simulink model "asbQuadcopter"  (R2018b)
settings: Solver=ode3  StartTime=0  StopTime=TFinal  FixedStep=Ts  RelTol=1e-3  EnableMultiTasking=on
undefined symbols (not defined in the file or in its folder): Command, ft, init, m, s, takeOffDuration, Ts, Vehicle
libraries: simulink x16, aerolibconvert2 x4, aerolibanimutils x2, SignalEditorBlockLib x2, environmentLibrary x2, sensorsLibrary x2, aerolibfltsims x2, aerolibutil x2, vrlib x1
settings Model: Creator=The MathWorks, Inc.  LastModifiedBy=The MathWorks, Inc.
settings DataIOCC: LimitDataPoints=on  SaveFormat=Array  SaveOutput=off  SignalLogging=off  DSMLogging=off  SaveTime=off
settings OptimizationCC: BlockReduction=off  BufferReuse=off  LifeSpan=inf
settings DebuggingCC: AlgebraicLoopMsg=none  ParameterPrecisionLossMsg=none  UnconnectedInputMsg=none  UnconnectedOutputMsg=none  UnconnectedLineMsg=none  AllowSymbolicDim=off  LibraryContextMissingDiagnostic=none  SFUnexpectedBacktrackingDiag=warning  SFNoUnconditionalDefaultTransitionDiag=warning  SFExecutionAtInitializationDiag=none
settings HardwareCC: ProdBitPerPointer=32  ProdBitPerSizeT=32  ProdBitPerPtrDiffT=32  ProdLargestAtomicFloat=None  ProdIntDivRoundTo=Undefined  ProdEndianess=Unspecified  ProdWordSize=32  ProdHWDeviceType=32-bit Generic
settings ModelReferenceCC: PropagateSignalLabelsOutOfModel=off
settings SFSimCC: SimUseLocalCustomCode=off
settings RTWCC: RTWUseLocalCustomCode=off
settings CodeAppCC: StateflowObjectComments=on
settings GRTTargetCC: TargetLangStandard=C89/C90 (ANSI)  GeneratePreprocessorConditionals=Disable all
settings ConfigComp: CovMetricSettings=dw  CovHtmlReporting=on  CovSaveCumulativeToWorkspaceVar=on  CovSaveSingleToWorkspaceVar=on  CovExternalEMLEnable=off  CovSFcnEnable=off

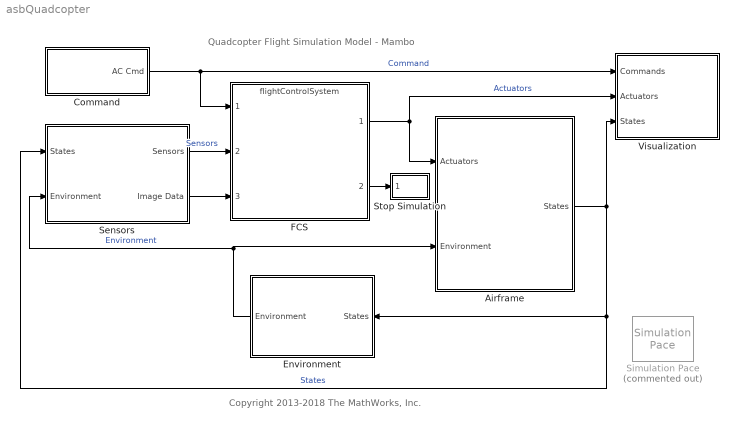
== system asbQuadcopter ==
  note: Quadcopter Flight Simulation Model - Mambo
  note: Copyright 2013-2018 The MathWorks, Inc.
  Airframe : Subsystem  Variant=on
  Command : Subsystem  Variant=on
  Environment : Subsystem  Variant=on
  FCS : ModelReference  ModelNameDialog=flightControlSystem.slx  SimulationMode=Normal  ModelReferenceVersion=1.137
  Sensors : Subsystem  Variant=on
  Simulation Pace : aerolibanimutils/Simulation Pace  Commented=on  SimulationPace=1  SleepMode=MATLAB Thread  OutputPaceError=off  SampleTime=Ts
      settings: AttributesFormatString=%<SimulationPace> sec/sec
  Stop Simulation : Subsystem
  Visualization : Subsystem
  wires:
  Command/1(AC Cmd) -> Visualization/1(Commands), FCS/1  "Command"
  Sensors/1(Sensors) -> FCS/2  "Sensors"
  FCS/1 -> Visualization/2(Actuators), Airframe/1(Actuators)  "Actuators"
  Environment/1(Environment) -> Airframe/2(Environment), Sensors/2(Environment)  "Environment"
  Airframe/1(States) -> Visualization/3(States), Environment/1(States), Sensors/1(States)  "States"
  FCS/2 -> Stop Simulation/1(Flags)
  Sensors/2(Image Data) -> FCS/3

== system asbQuadcopter/Airframe ==
  note: VSS_VEHICLE = 0 will select linear airframe
      | VSS_VEHICLE = 1 will select nonlnear airframe
  Actuators : Inport
  Environment : Inport  Port=2  OutDataTypeStr=Bus: EnvironmentBus
  Linear Airframe : ModelReference  ModelNameDialog=linearAirframe.slx  SimulationMode=Normal  VariantControl=VSS_VEHICLE_LINEAR  ModelReferenceVersion=1.39
  Nonlinear Airframe : ModelReference  ModelNameDialog=nonlinearAirframe.slx  SimulationMode=Normal  VariantControl=VSS_VEHICLE_NONLINEAR  ModelReferenceVersion=1.149
  States : Outport  OutDataTypeStr=Bus: StatesBus

== system asbQuadcopter/Command ==
  note: VSS_COMMAND = 0 will select Signal Editor
      | VSS_COMMAND = 1 will select Joystick + Signal Editor
      | VSS_COMMAND = 2 will select pre-saved data from .mat file
      | VSS_COMMAND = 3 will select pre-saved data from a spreadsheet
  Data : Subsystem  VariantControl=VSS_COMMAND_PRESAVED
  Joystick : Subsystem  VariantControl=VSS_COMMAND_JOYSTICK
  Signal Editor : Subsystem  VariantControl=VSS_COMMAND_SIGEDIT
  Spreadsheet Data : Subsystem  VariantControl=VSS_COMMAND_SPREADSHEET
  AC Cmd : Outport  OutDataTypeStr=Bus: CommandBus

== system asbQuadcopter/Environment ==
  note: VSS_ENVIRONMENT = 0 will select constant environment variables
      | VSS_ENVIRONMENT = 1 will select environment variables depending on position
  States : Inport  OutDataTypeStr=Bus: StatesBus
  Environment (Constant) : environmentLibrary/Environment (Constant)  SystemSampleTime=-1  VariantControl=VSS_ENVIRONMENT_CST
      settings: SourceProductName=Aerospace Blockset  SourceProductBaseCode=AE
  Environment (Variable) : environmentLibrary/Environment (Variable)  SystemSampleTime=-1  VariantControl=VSS_ENVIRONMENT_VARIABLE
      settings: SourceProductName=Aerospace Blockset  SourceProductBaseCode=AE
  Environment : Outport  OutDataTypeStr=Bus: EnvironmentBus

== system asbQuadcopter/Sensors ==
  note: VSS_SENSORS = 0 will select feedthrough sensors
      | VSS_SENSORS = 1 will select dynamics sensors with noise
  States : Inport
  Environment : Inport  Port=2
  Sensors (Dynamics) : sensorsLibrary/Sensors (Dynamics)  SystemSampleTime=-1  VariantControl=VSS_SENSORS_DYNAMICS
      settings: SourceProductName=Aerospace Blockset  SourceProductBaseCode=AE
  Sensors (Feedthrough) : sensorsLibrary/Sensors (Feedthrough)  SystemSampleTime=-1  VariantControl=VSS_SENSORS_FEEDTHROUGH
      settings: SourceProductName=Aerospace Blockset  SourceProductBaseCode=AE
  Sensors : Outport
  Image Data : Outport  Port=2

== system asbQuadcopter/Stop Simulation ==
  Flags : Inport  OutDataTypeStr=uint8
  Compare To Zero : simulink/Logic and Bit Operations/Compare To Zero  relop=>  OutDataTypeStr=boolean
  Flag has been triggered : Assertion
  Logical Operator : Logic  Operator=NOT  AllPortsSameDT=off  OutDataTypeStr=boolean
  wires:
  Flags/1 -> Compare To Zero/1
  Logical Operator/1 -> Flag has been triggered/1
  Compare To Zero/1 -> Logical Operator/1

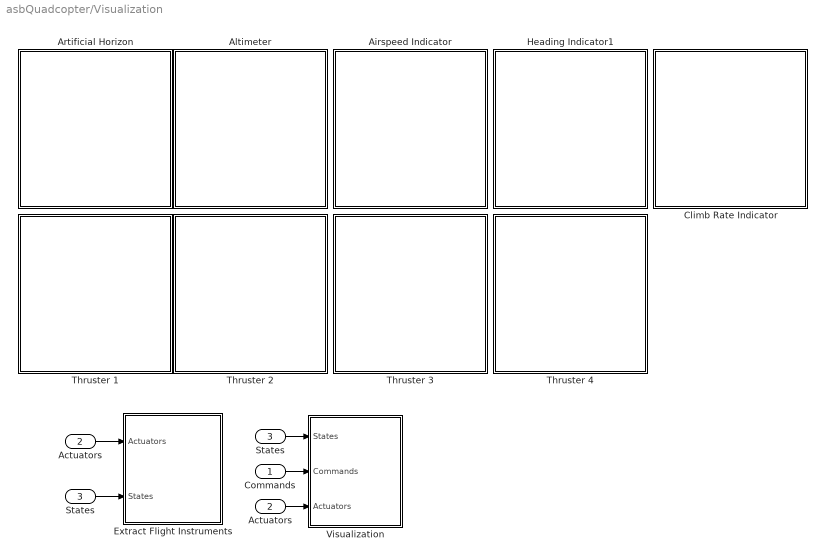
== system asbQuadcopter/Visualization ==
  Commands : Inport
  Actuators : Inport  Port=2
  States : Inport  Port=3
  "Actuators " : InportShadow  Port=2
  Airspeed Indicator : Subsystem  DialogController=aeroblksHMICreateDDGDialog  IsWebBlock=on  mask(MWDashboardBlock){webBlockId=18ef8fab-31e9-4f7d-84d7-de450e3677f8, webBlockType=airspeedindicator, ShowLibInBrowser=on, ShowInitialText=on, HMISrcModelName=asbQuadcopter}
      mask prompts: webBlockId "WebBlock Id"; webBlockType "WebBlock Type"; HMISrcModelName "Source Model"
      mask help: aeroblksHMI:aeroblkhmi:AirspeedIndicatorDialogDesc
      mask Help: eval('asbhmihelp(''airspeedindicator'')');
      mask Display:
      | if strcmp(get_param(bdroot(gcb),'BlockDiagramType'), 'library')
      |  image([(matlabroot) '/toolbox/aeroblks/aeroblks/hmi/icons/AirspeedIndicatorIcon.svg'])
      | end
  Altimeter : Subsystem  DialogController=aeroblksHMICreateDDGDialog  IsWebBlock=on  mask(MWDashboardBlock){webBlockId=100f33d8-dd26-4cf5-9a56-796be033f673, webBlockType=altimeter, ShowLibInBrowser=on, ShowInitialText=on, HMISrcModelName=asbQuadcopter}
      mask prompts: webBlockId "WebBlock Id"; webBlockType "WebBlock Type"; HMISrcModelName "Source Model"
      mask help: aeroblksHMI:aeroblkhmi:AltimeterDialogDesc
      mask Help: eval('asbhmihelp(''altimeter'')');
      mask Display:
      | if strcmp(get_param(bdroot(gcb),'BlockDiagramType'), 'library')
      |  image([(matlabroot) '/toolbox/aeroblks/aeroblks/hmi/icons/AltimeterIcon.svg'])
      | end
  Artificial Horizon : Subsystem  DialogController=aeroblksHMICreateDDGDialog  IsWebBlock=on  mask(MWDashboardBlock){webBlockId=2f185b59-f257-45c3-93d6-8e4e2ebb9412, webBlockType=artificialhorizon, ShowLibInBrowser=on, ShowInitialText=on, HMISrcModelName=asbQuadcopter}
      mask prompts: webBlockId "WebBlock Id"; webBlockType "WebBlock Type"; HMISrcModelName "Source Model"
      mask help: aeroblksHMI:aeroblkhmi:ArtificialHorizonDialogDesc
      mask Help: eval('asbhmihelp(''artificialhorizon'')');
      mask Display:
      | if strcmp(get_param(bdroot(gcb),'BlockDiagramType'), 'library')
      |  image([(matlabroot) '/toolbox/aeroblks/aeroblks/hmi/icons/ArtificialHorizonIcon.svg'])
      | end
  Climb Rate Indicator : Subsystem  DialogController=aeroblksHMICreateDDGDialog  IsWebBlock=on  mask(MWDashboardBlock){webBlockId=01b27fea-40d1-4afa-95b8-217bdf758396, webBlockType=climbindicator, ShowLibInBrowser=on, ShowInitialText=on, HMISrcModelName=asbQuadcopter}
      mask prompts: webBlockId "WebBlock Id"; webBlockType "WebBlock Type"; HMISrcModelName "Source Model"
      mask Help: eval('asbhmihelp(''climbindicator'')');
      mask Display:
      | if strcmp(get_param(bdroot(gcb),'BlockDiagramType'), 'library')
      |  image([(matlabroot) '/toolbox/aeroblks/aeroblks/hmi/icons/ClimbIndicatorIcon.svg'])
      | end
  Extract Flight Instruments : Subsystem
  Heading Indicator1 : Subsystem  DialogController=aeroblksHMICreateDDGDialog  IsWebBlock=on  mask(MWDashboardBlock){webBlockId=349a9895-ae71-4c34-aaf3-8a4b044263fc, webBlockType=headingindicator, ShowLibInBrowser=on, ShowInitialText=on, HMISrcModelName=asbQuadcopter}
      mask prompts: webBlockId "WebBlock Id"; webBlockType "WebBlock Type"; HMISrcModelName "Source Model"
      mask help: aeroblksHMI:aeroblkhmi:HeadingIndicatorDialogDesc
      mask Help: eval('asbhmihelp(''headingindicator'')');
      mask Display:
      | if strcmp(get_param(bdroot(gcb),'BlockDiagramType'), 'library')
      |  image([(matlabroot) '/toolbox/aeroblks/aeroblks/hmi/icons/HeadingIndicatorIcon.svg'])
      | end
  "States " : InportShadow  Port=3
  Thruster 1 : Subsystem  DialogController=aeroblksHMICreateDDGDialog  IsWebBlock=on  mask(MWDashboardBlock){webBlockId=cb5b89b4-9a60-4ffc-8d4b-680aac62b0ad, webBlockType=rpmindicator, ShowLibInBrowser=on, ShowInitialText=on, HMISrcModelName=asbQuadcopter}
      mask prompts: webBlockId "WebBlock Id"; webBlockType "WebBlock Type"; HMISrcModelName "Source Model"
      mask help: aeroblksHMI:aeroblkhmi:RPMIndicatorDialogDesc
      mask Help: eval('asbhmihelp(''rpmindicator'')')
      mask Display:
      | if strcmp(get_param(bdroot(gcb),'BlockDiagramType'), 'library')
      |  image([(matlabroot) '/toolbox/aeroblks/aeroblks/hmi/icons/RPMIndicatorIcon.svg'])
      | end
  Thruster 2 : Subsystem  DialogController=aeroblksHMICreateDDGDialog  IsWebBlock=on  mask(MWDashboardBlock){webBlockId=f0cf643f-3686-4bab-9794-ec5ca9f0526b, webBlockType=rpmindicator, ShowLibInBrowser=on, ShowInitialText=on, HMISrcModelName=asbQuadcopter}
      mask prompts: webBlockId "WebBlock Id"; webBlockType "WebBlock Type"; HMISrcModelName "Source Model"
      mask help: aeroblksHMI:aeroblkhmi:RPMIndicatorDialogDesc
      mask Help: eval('asbhmihelp(''rpmindicator'')')
      mask Display:
      | if strcmp(get_param(bdroot(gcb),'BlockDiagramType'), 'library')
      |  image([(matlabroot) '/toolbox/aeroblks/aeroblks/hmi/icons/RPMIndicatorIcon.svg'])
      | end
  Thruster 3 : Subsystem  DialogController=aeroblksHMICreateDDGDialog  IsWebBlock=on  mask(MWDashboardBlock){webBlockId=fde82f48-64f7-4e22-ac0c-568ccc998d28, webBlockType=rpmindicator, ShowLibInBrowser=on, ShowInitialText=on, HMISrcModelName=asbQuadcopter}
      mask prompts: webBlockId "WebBlock Id"; webBlockType "WebBlock Type"; HMISrcModelName "Source Model"
      mask help: aeroblksHMI:aeroblkhmi:RPMIndicatorDialogDesc
      mask Help: eval('asbhmihelp(''rpmindicator'')')
      mask Display:
      | if strcmp(get_param(bdroot(gcb),'BlockDiagramType'), 'library')
      |  image([(matlabroot) '/toolbox/aeroblks/aeroblks/hmi/icons/RPMIndicatorIcon.svg'])
      | end
  Thruster 4 : Subsystem  DialogController=aeroblksHMICreateDDGDialog  IsWebBlock=on  mask(MWDashboardBlock){webBlockId=9efa2ed4-730f-4ead-a19e-56fcb1fb4e55, webBlockType=rpmindicator, ShowLibInBrowser=on, ShowInitialText=on, HMISrcModelName=asbQuadcopter}
      mask prompts: webBlockId "WebBlock Id"; webBlockType "WebBlock Type"; HMISrcModelName "Source Model"
      mask help: aeroblksHMI:aeroblkhmi:RPMIndicatorDialogDesc
      mask Help: eval('asbhmihelp(''rpmindicator'')')
      mask Display:
      | if strcmp(get_param(bdroot(gcb),'BlockDiagramType'), 'library')
      |  image([(matlabroot) '/toolbox/aeroblks/aeroblks/hmi/icons/RPMIndicatorIcon.svg'])
      | end
  Visualization : Subsystem  Variant=on
  wires:
  Actuators/1 -> Extract Flight Instruments/1(Actuators)
  States/1 -> Extract Flight Instruments/2(States)
  Commands/1 -> Visualization/2(Commands)
  "Actuators "/1 -> Visualization/3(Actuators)
  "States "/1 -> Visualization/1(States)

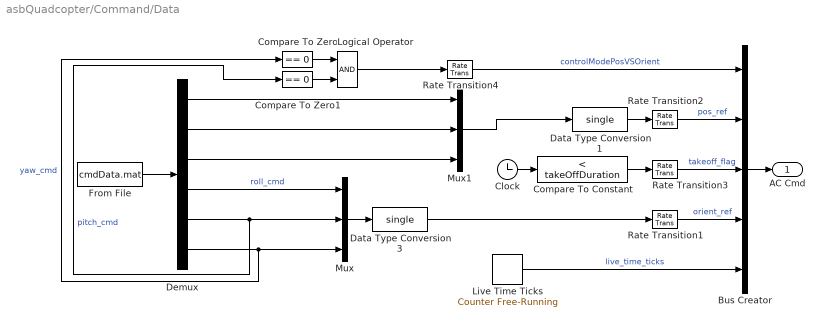
== system asbQuadcopter/Command/Data ==
  Bus Creator : BusCreator  Inputs=5  OutDataTypeStr=Bus: CommandBus  NonVirtualBus=on
  Clock : Clock
  Compare To Constant : simulink/Logic and Bit Operations/Compare To Constant  relop=<  const=takeOffDuration  OutDataTypeStr=boolean
  Compare To Zero : simulink/Logic and Bit Operations/Compare To Zero  relop===  OutDataTypeStr=boolean
  Compare To Zero1 : simulink/Logic and Bit Operations/Compare To Zero  relop===  OutDataTypeStr=boolean
  Data Type Conversion1 : DataTypeConversion  OutDataTypeStr=single
  Data Type Conversion3 : DataTypeConversion  OutDataTypeStr=single
  Demux : Demux  Outputs=6
  From File : FromFile  FileName=cmdData.mat  SampleTime=Ts
  Live Time Ticks : simulink/Sources/Counter Free-Running  NumBits=32  tsamp=Ts
  Logical Operator : Logic  IconShape=distinctive  AllPortsSameDT=off  OutDataTypeStr=boolean
  Mux : Mux  Inputs=3
  Mux1 : Mux  Inputs=3
  Rate Transition{1..4} (4 alike) : RateTransition  OutPortSampleTime=Ts
  AC Cmd : Outport  OutDataTypeStr=Bus: CommandBus
  wires:
  Demux/4 -> Mux/1  "roll_cmd"
  Demux/5 -> Mux/2, Compare To Zero1/1  "pitch_cmd"
  Demux/6 -> Compare To Zero/1, Mux/3  "yaw_cmd"
  From File/1 -> Demux/1
  Logical Operator/1 -> Rate Transition4/1
  Rate Transition1/1 -> Bus Creator/4  "orient_ref"
  Rate Transition2/1 -> Bus Creator/2  "pos_ref"
  Demux/3 -> Mux1/3
  Mux/1 -> Data Type Conversion3/1
  Data Type Conversion1/1 -> Rate Transition2/1
  Demux/1 -> Mux1/1
  Compare To Zero1/1 -> Logical Operator/2
  Compare To Zero/1 -> Logical Operator/1
  Mux1/1 -> Data Type Conversion1/1
  Clock/1 -> Compare To Constant/1
  Rate Transition4/1 -> Bus Creator/1  "controlModePosVSOrient"
  Data Type Conversion3/1 -> Rate Transition1/1
  Demux/2 -> Mux1/2
  Compare To Constant/1 -> Rate Transition3/1
  Rate Transition3/1 -> Bus Creator/3  "takeoff_flag"
  Live Time Ticks/1 -> Bus Creator/5  "live_time_ticks"
  Bus Creator/1 -> AC Cmd/1

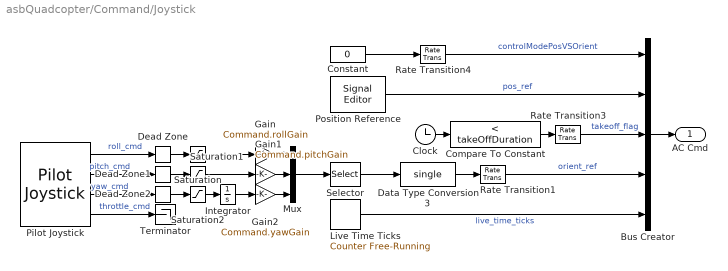
== system asbQuadcopter/Command/Joystick ==
  Bus Creator : BusCreator  Inputs=5  OutDataTypeStr=Bus: CommandBus  NonVirtualBus=on
  Clock : Clock
  Compare To Constant : simulink/Logic and Bit Operations/Compare To Constant  relop=<  const=takeOffDuration  OutDataTypeStr=boolean
  Constant : Constant  Value=0  OutDataTypeStr=boolean
  Data Type Conversion3 : DataTypeConversion  OutDataTypeStr=single
  Dead Zone : DeadZone  LowerValue=Command.rollDeadZoneStart  UpperValue=Command.rollDeadZoneEnd  SaturateOnIntegerOverflow=on
  Dead Zone1 : DeadZone  LowerValue=Command.pitchDeadZoneStart  UpperValue=Command.pitchDeadZoneEnd  SaturateOnIntegerOverflow=on
  Dead Zone2 : DeadZone  LowerValue=Command.yawDeadZoneStart  UpperValue=Command.yawDeadZoneEnd  SaturateOnIntegerOverflow=on
  Gain : Gain  Gain=Command.rollGain
  Gain1 : Gain  Gain=Command.pitchGain
  Gain2 : Gain  Gain=Command.yawGain
  Integrator : Integrator
  Live Time Ticks : simulink/Sources/Counter Free-Running  NumBits=32  tsamp=Ts
  Mux : Mux  Inputs=3
  Pilot Joystick : aerolibanimutils/Pilot Joystick  JoystickID=Joystick1  OutputConfiguration=FourAxis  SampleTime=Ts
  Position Reference : SignalEditorBlockLib/Signal Editor  FileName=positionRef.mat  ActiveScenario=Group1  ActiveSignal=XYZ  IsBus=off  OutputBusObjectStr=Bus: BusObject  SampleTime=Ts  Interpolate=off  ZeroCross=off  OutputAfterFinalValue=Setting to zero  Unit=inherit
  Rate Transition1 : RateTransition  OutPortSampleTime=Ts
  Rate Transition3 : RateTransition  OutPortSampleTime=Ts
  Rate Transition4 : RateTransition  OutPortSampleTime=Ts
  Saturation : Saturate  UpperLimit=Command.rollSatUpper  LowerLimit=Command.rollSatLower
  Saturation1 : Saturate  UpperLimit=Command.pitchSatUpper  LowerLimit=Command.pitchSatLower
  Saturation2 : Saturate  UpperLimit=Command.yawSatUpper  LowerLimit=Command.yawSatLower
  Selector : Selector  InputPortWidth=3  IndexOptions=Index vector (dialog)  Indices=[3 2 1]  OutputSizes=1
  Terminator : Terminator
  AC Cmd : Outport  OutDataTypeStr=Bus: CommandBus
  wires:
  Pilot Joystick/4 -> Terminator/1  "throttle_cmd"
  Pilot Joystick/1 -> Dead Zone/1  "roll_cmd"
  Bus Creator/1 -> AC Cmd/1
  Constant/1 -> Rate Transition4/1
  Rate Transition1/1 -> Bus Creator/4  "orient_ref"
  Position Reference/1 -> Bus Creator/2  "pos_ref"
  Mux/1 -> Selector/1
  Compare To Constant/1 -> Rate Transition3/1
  Clock/1 -> Compare To Constant/1
  Rate Transition4/1 -> Bus Creator/1  "controlModePosVSOrient"
  Data Type Conversion3/1 -> Rate Transition1/1
  Pilot Joystick/2 -> Dead Zone1/1  "pitch_cmd"
  Rate Transition3/1 -> Bus Creator/3  "takeoff_flag"
  Live Time Ticks/1 -> Bus Creator/5  "live_time_ticks"
  Selector/1 -> Data Type Conversion3/1
  Dead Zone/1 -> Saturation/1
  Saturation/1 -> Gain/1
  Gain/1 -> Mux/1
  Dead Zone1/1 -> Saturation1/1
  Saturation1/1 -> Gain1/1
  Gain1/1 -> Mux/2
  Dead Zone2/1 -> Saturation2/1
  Saturation2/1 -> Integrator/1
  Gain2/1 -> Mux/3
  Pilot Joystick/3 -> Dead Zone2/1  "yaw_cmd"
  Integrator/1 -> Gain2/1

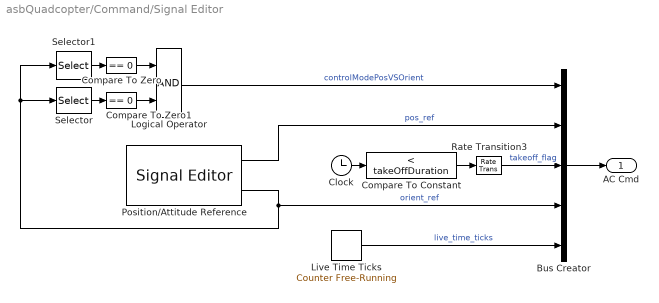
== system asbQuadcopter/Command/Signal Editor ==
  Bus Creator : BusCreator  Inputs=5  OutDataTypeStr=Bus: CommandBus  NonVirtualBus=on
  Clock : Clock
  Compare To Constant : simulink/Logic and Bit Operations/Compare To Constant  relop=<  const=takeOffDuration  OutDataTypeStr=boolean
  Compare To Zero : simulink/Logic and Bit Operations/Compare To Zero  relop===  OutDataTypeStr=boolean
  Compare To Zero1 : simulink/Logic and Bit Operations/Compare To Zero  relop===  OutDataTypeStr=boolean
  Live Time Ticks : simulink/Sources/Counter Free-Running  NumBits=32  tsamp=Ts
  Logical Operator : Logic  AllPortsSameDT=off  OutDataTypeStr=boolean
  Position/Attitude Reference : SignalEditorBlockLib/Signal Editor  FileName=positionAttitudeRef.mat  ActiveScenario=Hover  ActiveSignal=XYZ  IsBus=off  OutputBusObjectStr=Bus: BusObject  SampleTime=Ts  Interpolate=off  ZeroCross=off  OutputAfterFinalValue=Holding final value  Unit=inherit
  Rate Transition3 : RateTransition  OutPortSampleTime=Ts
  Selector : Selector  InputPortWidth=3  IndexOptions=Index vector (dialog)  Indices=2  OutputSizes=1
  Selector1 : Selector  InputPortWidth=3  IndexOptions=Index vector (dialog)  Indices=3  OutputSizes=1
  AC Cmd : Outport  OutDataTypeStr=Bus: CommandBus
  wires:
  Bus Creator/1 -> AC Cmd/1
  Position/Attitude Reference/2 -> Bus Creator/4, Selector1/1, Selector/1  "orient_ref"
  Compare To Zero/1 -> Logical Operator/1
  Compare To Zero1/1 -> Logical Operator/2
  Logical Operator/1 -> Bus Creator/1  "controlModePosVSOrient"
  Position/Attitude Reference/1 -> Bus Creator/2  "pos_ref"
  Clock/1 -> Compare To Constant/1
  Compare To Constant/1 -> Rate Transition3/1
  Rate Transition3/1 -> Bus Creator/3  "takeoff_flag"
  Live Time Ticks/1 -> Bus Creator/5  "live_time_ticks"
  Selector/1 -> Compare To Zero1/1
  Selector1/1 -> Compare To Zero/1

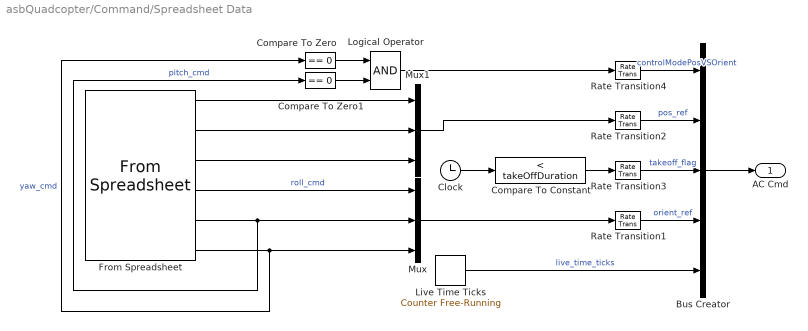
== system asbQuadcopter/Command/Spreadsheet Data ==
  Bus Creator : BusCreator  Inputs=5  OutDataTypeStr=Bus: CommandBus  NonVirtualBus=on
  Clock : Clock
  Compare To Constant : simulink/Logic and Bit Operations/Compare To Constant  relop=<  const=takeOffDuration  OutDataTypeStr=boolean
  Compare To Zero : simulink/Logic and Bit Operations/Compare To Zero  relop===  OutDataTypeStr=boolean
  Compare To Zero1 : simulink/Logic and Bit Operations/Compare To Zero  relop===  OutDataTypeStr=boolean
  From Spreadsheet : FromSpreadsheet  FileName=cmdData.xlsx  SheetName=data  OutDataTypeStr=single  SampleTime=Ts
  Live Time Ticks : simulink/Sources/Counter Free-Running  NumBits=32  tsamp=Ts
  Logical Operator : Logic  IconShape=distinctive  AllPortsSameDT=off  OutDataTypeStr=boolean
  Mux : Mux  Inputs=3
  Mux1 : Mux  Inputs=3
  Rate Transition{1..4} (4 alike) : RateTransition  OutPortSampleTime=Ts
  AC Cmd : Outport  OutDataTypeStr=Bus: CommandBus
  wires:
  Bus Creator/1 -> AC Cmd/1
  From Spreadsheet/4 -> Mux/1  "roll_cmd"
  From Spreadsheet/6 -> Mux/3, Compare To Zero/1  "yaw_cmd"
  Logical Operator/1 -> Rate Transition4/1
  Rate Transition1/1 -> Bus Creator/4  "orient_ref"
  Rate Transition2/1 -> Bus Creator/2  "pos_ref"
  From Spreadsheet/3 -> Mux1/3
  Mux1/1 -> Rate Transition2/1
  From Spreadsheet/1 -> Mux1/1
  Compare To Zero1/1 -> Logical Operator/2
  Compare To Zero/1 -> Logical Operator/1
  Compare To Constant/1 -> Rate Transition3/1
  Clock/1 -> Compare To Constant/1
  Rate Transition4/1 -> Bus Creator/1  "controlModePosVSOrient"
  Mux/1 -> Rate Transition1/1
  From Spreadsheet/5 -> Mux/2, Compare To Zero1/1  "pitch_cmd"
  From Spreadsheet/2 -> Mux1/2
  Rate Transition3/1 -> Bus Creator/3  "takeoff_flag"
  Live Time Ticks/1 -> Bus Creator/5  "live_time_ticks"

== system asbQuadcopter/Visualization/Airspeed Indicator ==

== system asbQuadcopter/Visualization/Altimeter ==

== system asbQuadcopter/Visualization/Artificial Horizon ==

== system asbQuadcopter/Visualization/Climb Rate Indicator ==

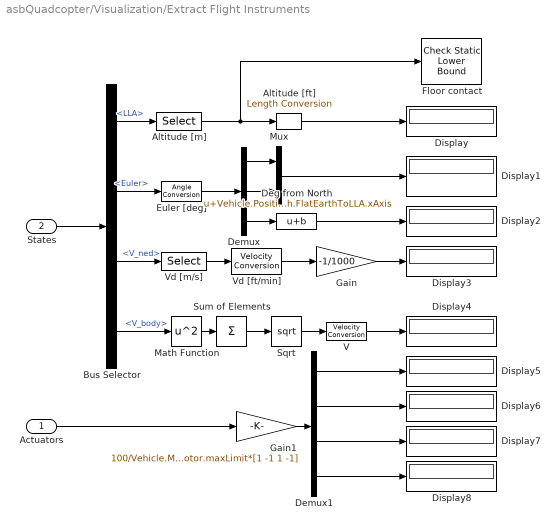
== system asbQuadcopter/Visualization/Extract Flight Instruments ==
  Actuators : Inport
  States : Inport  Port=2
  Altitude [ft] : aerolibconvert2/Length Conversion  IU=m  OU=ft
  Altitude [m] : Selector  InputPortWidth=3  IndexOptions=Index vector (dialog)  Indices=[3]  OutputSizes=1
  Bus Selector : BusSelector  OutputSignals=LLA,Euler,V_ned,V_body
  Deg from North : Bias  Bias=Vehicle.PositionOnEarth.FlatEarthToLLA.xAxis
  Demux : Demux  Outputs=3
  Demux1 : Demux
  Display{,1..8} (9 alike) : Display
  Euler [deg] : aerolibconvert2/Angle Conversion  IU=rad  OU=deg
  Floor contact : simulink/Model Verification/Check Static  Lower Bound  Description=init.posLLA(3) <= u  min=init.posLLA(3)  min_included=on  enabled=on  stopWhenAssertionFail=on  export=off  icon=graphic
      settings: SourceProductName=Simulink
  Gain : Gain  Gain=-1/1000
  Gain1 : Gain  Gain=100/Vehicle.Motor.maxLimit*[1 -1 1 -1]
  Math Function : Math  Operator=square  SaturateOnIntegerOverflow=on
  Mux : Mux  Inputs=2
  Sqrt : Sqrt  SaturateOnIntegerOverflow=on
  Sum of Elements : Sum  Inputs=+
  V : aerolibconvert2/Velocity Conversion  IU=m/s  OU=kts
  Vd [ft/min] : aerolibconvert2/Velocity Conversion  IU=m/s  OU=ft/min
  Vd [m/s] : Selector  InputPortWidth=3  IndexOptions=Index vector (dialog)  Indices=[3]  OutputSizes=1
  wires:
  Bus Selector/1 -> Altitude [m]/1  "<LLA>"
  Altitude [m]/1 -> Floor contact/1, Altitude [ft]/1
  States/1 -> Bus Selector/1
  Altitude [ft]/1 -> Display/1
  Bus Selector/2 -> Euler [deg]/1  "<Euler>"
  Euler [deg]/1 -> Demux/1
  Demux/1 -> Mux/1
  Demux/2 -> Mux/2
  Mux/1 -> Display1/1
  Deg from North/1 -> Display2/1
  Bus Selector/3 -> Vd [m/s]/1  "<V_ned>"
  Vd [m/s]/1 -> Vd [ft/min]/1
  Vd [ft/min]/1 -> Gain/1
  Gain/1 -> Display3/1
  Math Function/1 -> Sum of Elements/1
  Sum of Elements/1 -> Sqrt/1
  Bus Selector/4 -> Math Function/1  "<V_body>"
  Sqrt/1 -> V/1
  V/1 -> Display4/1
  Gain1/1 -> Demux1/1
  Demux1/1 -> Display5/1
  Demux1/2 -> Display6/1
  Demux1/3 -> Display7/1
  Demux1/4 -> Display8/1
  Actuators/1 -> Gain1/1
  Demux/3 -> Deg from North/1

== system asbQuadcopter/Visualization/Heading Indicator1 ==

== system asbQuadcopter/Visualization/Thruster 1 ==

== system asbQuadcopter/Visualization/Thruster 2 ==

== system asbQuadcopter/Visualization/Thruster 3 ==

== system asbQuadcopter/Visualization/Thruster 4 ==

== system asbQuadcopter/Visualization/Visualization ==
  note: VSS_VISUALIZATION = 0 will select scopes as means to visualie variables/states
      | VSS_VISUALIZATION = 1 will send select states in a variable to the workspace
      | VSS_VISUALIZATION = 2 will use FlightGear as visualization
      | VSS_VISUALIZATION = 3 will use a Simulink 3D interface
  States : Inport  OutDataTypeStr=Bus: StatesBus
  Commands : Inport  Port=2  OutDataTypeStr=Bus: CommandBus
  Actuators : Inport  Port=3
  FlightGear : Subsystem  VariantControl=VSS_VISUALIZATION_FLIGHTGEAR
      mask init:
      | visualizationFlightGearVars;
  Scopes : Subsystem  VariantControl=VSS_VISUALIZATION_SCOPES
  Simulink 3D : Subsystem  VariantControl=VSS_VISUALIZATION_SL3D
      mask init:
      | visualizationFlightGearVars;
  Workspace : Subsystem  VariantControl=VSS_VISUALIZATION_WORKSPACE

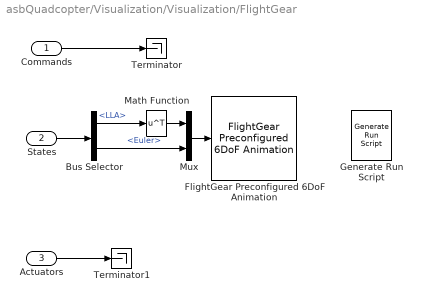
== system asbQuadcopter/Visualization/Visualization/FlightGear ==
  Commands : Inport
  States : Inport  Port=2
  Actuators : Inport  Port=3
  Bus Selector : BusSelector  OutputSignals=LLA,Euler
  FlightGear Preconfigured 6DoF Animation : aerolibfltsims/FlightGear Preconfigured 6DoF Animation  xFlightGearVersion=v2017.3  DestinationIpAddress=127.0.0.1  DestinationPort=Visualization.FlightGear.SixDOF.destinationPort  SampleTime=Ts
      settings: SourceProductName=Aerospace Blockset
  Generate Run Script : aerolibfltsims/Generate Run Script  Architecture=Default  dataFlow=Send  GeometryModelName=Model  AirportId=KSFO  RunwayId=10L  InitialAltitude=Visualization.FlightGear.generateRunScript.initialAltitude  InitialHeading=Visualization.FlightGear.generateRunScript.initialHeading  OffsetDistance=Visualization.FlightGear.generateRunScript.offsetDistance  OffsetAzimuth=Visualization.FlightGear.generateRunScript.offsetAzimuth  InstallScenery=off  DisableShaders=off  OriginAddress=127.0.0.1  DestinationPort=Visualization.FlightGear.generateRunScript.destinationPort  OriginPort=5505  LocalAddress=127.0.0.1  OutputFileName=runfg.bat  FlightGearBaseDirectory=C:\Program Files\FlightGear
  Math Function : Math  Operator=transpose  SaturateOnIntegerOverflow=on
  Mux : Mux  Inputs=2
  Terminator : Terminator
  Terminator1 : Terminator
  wires:
  States/1 -> Bus Selector/1
  Bus Selector/2 -> Mux/2  "<Euler>"
  Mux/1 -> FlightGear Preconfigured 6DoF Animation/1
  Commands/1 -> Terminator/1
  Actuators/1 -> Terminator1/1
  Bus Selector/1 -> Math Function/1  "<LLA>"
  Math Function/1 -> Mux/1

== system asbQuadcopter/Visualization/Visualization/Scopes ==
  Commands : Inport
  States : Inport  Port=2
  Actuators : Inport  Port=3
  Bus Creator : BusCreator  Inputs=2
  Bus Selector : BusSelector  OutputSignals=States.V_body,States.Euler,States.X_ned
  Euler : Scope
  Terminator1 : Terminator
  V_body : Scope
  X_ned : Scope
  wires:
  Commands/1 -> Bus Creator/1  "Commands"
  States/1 -> Bus Creator/2  "States"
  Bus Creator/1 -> Bus Selector/1
  Bus Selector/1 -> V_body/1  "<V_body>"
  Bus Selector/2 -> Euler/1  "<Euler>"
  Bus Selector/3 -> X_ned/1  "<X_ned>"
  Actuators/1 -> Terminator1/1

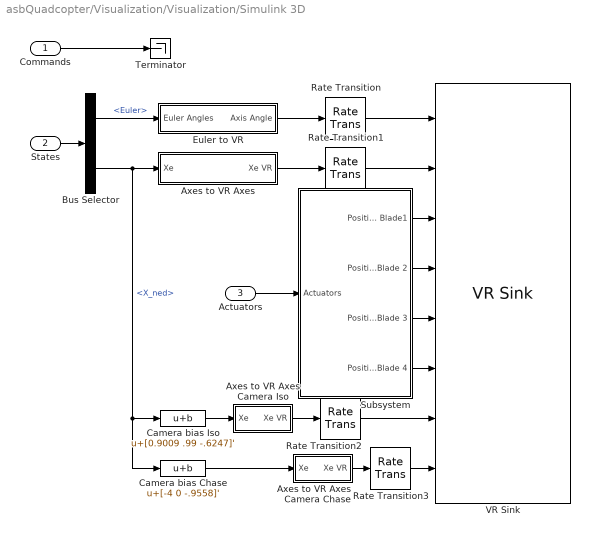
== system asbQuadcopter/Visualization/Visualization/Simulink 3D ==
  Commands : Inport
  States : Inport  Port=2
  Actuators : Inport  Port=3
  Axes to VR Axes : Subsystem
  Axes to VR Axes Camera Chase : Subsystem
  Axes to VR Axes Camera Iso : Subsystem
  Bus Selector : BusSelector  OutputSignals=Euler,X_ned
  Camera bias Chase : Bias  Bias=[-4 0 -.9558]'
  Camera bias Iso : Bias  Bias=[0.9009 .99 -.6247]'
  Euler to VR : Subsystem
  Rate Transition{,1..3} (4 alike) : RateTransition
  Subsystem : Subsystem
  Terminator : Terminator
  VR Sink : vrlib/VR Sink  InstantiateOnLoad=on  SampleTime=12*Ts  ViewEnable=on  RemoteChange=off  RemoteView=off  FieldsWritten=QuadBody.rotation.4.1.1.double#QuadBody.translation.3.1.1.double#Blade1.rotation.4.1.1.double#Blade3.rotation.4.1.1.double#Blade2.rotation.4.1.1.double#Blade4.rotation.4.1.1.double#IsoNoRotation.position.3.1.1.double#OnQuadNoRotation.position.3.1.1.double  WorldFileName=asbQuadcopterWorld.wrl  AutoView=on  VideoDimensions=[]  AllowVariableSize=off  FigureProperties="{'Position', 'Name', 'Viewpoint', 'CameraBound', 'CameraDirection', 'CameraPosition', 'CameraUpVector', 'ZoomFactor', 'Antialiasing', 'Headlight', 'Lighting', 'NavPanel', 'Sound', 'StatusBar', 'Stereo3D', 'Stereo3DCameraOffset', 'Stereo3DHIT', 'ToolBar', 'Textures', 'Transparency', 'Triad', 'Wireframe', 'NavZones', 'NavMode', 'NavSpeed', 'CaptureFileFormat', 'CaptureFileName', 'Record2DCompressMethod', 'Record2DCompressQuality', 'Record2D', 'Record2DFileName', 'Record2DFPS'; [5.0000000000000000e+00   1.0200000000000000e+02   5.7600000000000000e+02   3.5000000000000000e+02], '', 'Isometric', 'on', [0.0000000000000000e+00   0.0000000000000000e+00  -1.0000000000000000e+00], [0.0000000000000000e+00   0.0000000000000000e+00   0.0000000000000000e+00], [0.0000000000000000e+00   1.0000000000000000e+00   0.0000000000000000e+00], [1.0000000000000000e+00], 'on', 'on', 'on', 'halfbar', 'on', 'on', 'off', [1.0000000149011612e-01], [0.0000000000000000e+00], 'on', 'on', 'on', 'none', 'off', 'off', 'fly', 'normal', 'tif', '%f_anim_%n.tif', 'auto', [7.5000000000000000e+01], 'off', '%f_anim_%n.avi', 'auto'}"
      settings: SourceProductBaseCode=VR
  wires:
  Commands/1 -> Terminator/1
  Euler to VR/1(Axis Angle) -> Rate Transition/1
  Axes to VR Axes/1(Xe VR) -> Rate Transition1/1
  Bus Selector/1 -> Euler to VR/1(Euler Angles)  "<Euler>"
  Bus Selector/2 -> Camera bias Chase/1, Camera bias Iso/1, Axes to VR Axes/1(Xe)  "<X_ned>"
  States/1 -> Bus Selector/1
  Actuators/1 -> Subsystem/1(Actuators)
  Axes to VR Axes Camera Iso/1(Xe VR) -> Rate Transition2/1
  Camera bias Iso/1 -> Axes to VR Axes Camera Iso/1(Xe)
  Rate Transition/1 -> VR Sink/1
  Rate Transition1/1 -> VR Sink/2
  Subsystem/1(Position Blade1) -> VR Sink/3
  Subsystem/2(Position Blade 2) -> VR Sink/4
  Subsystem/3(Position Blade 3) -> VR Sink/5
  Subsystem/4(Position Blade 4) -> VR Sink/6
  Rate Transition2/1 -> VR Sink/7
  Axes to VR Axes Camera Chase/1(Xe VR) -> Rate Transition3/1
  Rate Transition3/1 -> VR Sink/8
  Camera bias Chase/1 -> Axes to VR Axes Camera Chase/1(Xe)

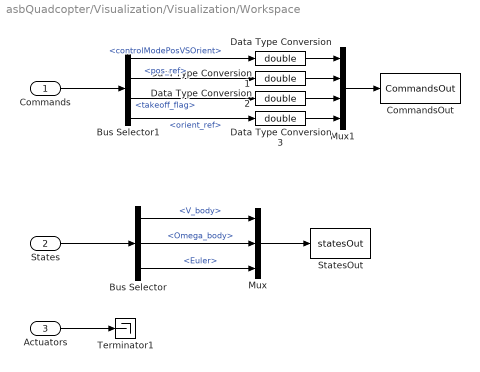
== system asbQuadcopter/Visualization/Visualization/Workspace ==
  Commands : Inport
  States : Inport  Port=2
  Actuators : Inport  Port=3
  Bus Selector : BusSelector  OutputSignals=V_body,Omega_body,Euler
  Bus Selector1 : BusSelector  OutputSignals=controlModePosVSOrient,pos_ref,takeoff_flag,orient_ref
  CommandsOut : ToWorkspace  VariableName=CommandsOut  SaveFormat=Structure With Time  SampleTime=-1
  Data Type Conversion{,1..3} (4 alike) : DataTypeConversion  OutDataTypeStr=double
  Mux : Mux  Inputs=3
  Mux1 : Mux
  StatesOut : ToWorkspace  VariableName=statesOut  SaveFormat=Structure With Time  SampleTime=-1
  Terminator1 : Terminator
  wires:
  States/1 -> Bus Selector/1
  Bus Selector/2 -> Mux/2  "<Omega_body>"
  Bus Selector/3 -> Mux/3  "<Euler>"
  Bus Selector/1 -> Mux/1  "<V_body>"
  Mux/1 -> StatesOut/1
  Commands/1 -> Bus Selector1/1
  Bus Selector1/2 -> Data Type Conversion1/1  "<pos_ref>"
  Bus Selector1/1 -> Data Type Conversion/1  "<controlModePosVSOrient>"
  Mux1/1 -> CommandsOut/1
  Bus Selector1/4 -> Data Type Conversion3/1  "<orient_ref>"
  Bus Selector1/3 -> Data Type Conversion2/1  "<takeoff_flag>"
  Actuators/1 -> Terminator1/1
  Data Type Conversion/1 -> Mux1/1
  Data Type Conversion1/1 -> Mux1/2
  Data Type Conversion2/1 -> Mux1/3
  Data Type Conversion3/1 -> Mux1/4

== system asbQuadcopter/Visualization/Visualization/Simulink 3D/Axes to VR Axes ==
  Xe : Inport
  Demux : Demux  Outputs=3
  Mux : Mux  Inputs=3
  rad-->deg1 : Gain  Gain=-1  SaturateOnIntegerOverflow=on  OutDataTypeStr=Inherit: Same as input  ParamDataTypeStr=Inherit: Same as input
  Xe VR : Outport
  wires:
  Xe/1 -> Demux/1
  Demux/1 -> Mux/1
  Demux/3 -> rad-->deg1/1
  Mux/1 -> Xe VR/1
  rad-->deg1/1 -> Mux/2
  Demux/2 -> Mux/3

== system asbQuadcopter/Visualization/Visualization/Simulink 3D/Axes to VR Axes Camera Chase ==
  Xe : Inport
  Demux : Demux  Outputs=3
  Mux : Mux  Inputs=3
  rad-->deg1 : Gain  Gain=-1  SaturateOnIntegerOverflow=on  OutDataTypeStr=Inherit: Same as input  ParamDataTypeStr=Inherit: Same as input
  Xe VR : Outport
  wires:
  Xe/1 -> Demux/1
  Demux/1 -> Mux/1
  Demux/3 -> rad-->deg1/1
  Mux/1 -> Xe VR/1
  rad-->deg1/1 -> Mux/2
  Demux/2 -> Mux/3

== system asbQuadcopter/Visualization/Visualization/Simulink 3D/Axes to VR Axes Camera Iso ==
  Xe : Inport
  Demux : Demux  Outputs=3
  Mux : Mux  Inputs=3
  rad-->deg1 : Gain  Gain=-1  SaturateOnIntegerOverflow=on  OutDataTypeStr=Inherit: Same as input  ParamDataTypeStr=Inherit: Same as input
  Xe VR : Outport
  wires:
  Demux/2 -> Mux/3
  rad-->deg1/1 -> Mux/2
  Mux/1 -> Xe VR/1
  Demux/3 -> rad-->deg1/1
  Demux/1 -> Mux/1
  Xe/1 -> Demux/1

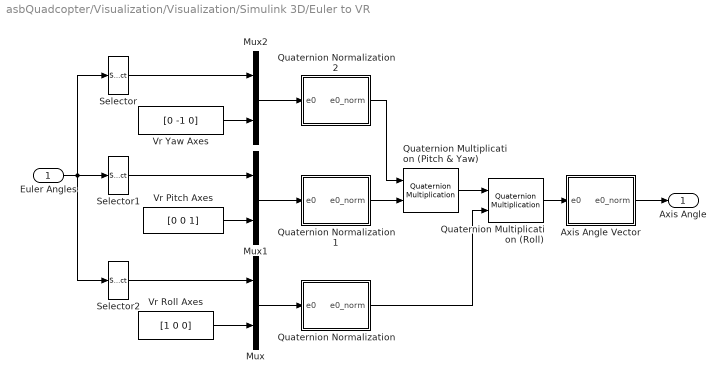
== system asbQuadcopter/Visualization/Visualization/Simulink 3D/Euler to VR ==
  Euler Angles : Inport
  Axis Angle Vector : Subsystem
  Mux : Mux  Inputs=2
  Mux1 : Mux  Inputs=2
  Mux2 : Mux  Inputs=2
  Quaternion Multiplication (Pitch & Yaw) : aerolibutil/Quaternion Multiplication
  Quaternion Multiplication (Roll) : aerolibutil/Quaternion Multiplication
  Quaternion Normalization : Subsystem
  Quaternion Normalization1 : Subsystem
  Quaternion Normalization2 : Subsystem
  Selector : Selector  InputPortWidth=3  IndexOptions=Index vector (dialog)  Indices=[3]  OutputSizes=1
  Selector1 : Selector  InputPortWidth=3  IndexOptions=Index vector (dialog)  Indices=[2]  OutputSizes=1
  Selector2 : Selector  InputPortWidth=3  IndexOptions=Index vector (dialog)  Indices=[1]  OutputSizes=1
  Vr Pitch Axes : Constant  Value=[0 0 1]
  Vr Roll Axes : Constant  Value=[1 0 0]
  Vr Yaw Axes : Constant  Value=[0 -1 0]
  Axis Angle : Outport
  wires:
  Quaternion Multiplication (Roll)/1 -> Axis Angle Vector/1(e0)
  Axis Angle Vector/1(e0_norm) -> Axis Angle/1
  Quaternion Normalization/1(e0_norm) -> Quaternion Multiplication (Roll)/2
  Quaternion Normalization2/1(e0_norm) -> Quaternion Multiplication (Pitch & Yaw)/1
  Quaternion Normalization1/1(e0_norm) -> Quaternion Multiplication (Pitch & Yaw)/2
  Mux2/1 -> Quaternion Normalization2/1(e0)
  Mux1/1 -> Quaternion Normalization1/1(e0)
  Mux/1 -> Quaternion Normalization/1(e0)
  Selector/1 -> Mux2/1
  Vr Yaw Axes/1 -> Mux2/2
  Selector1/1 -> Mux1/1
  Vr Pitch Axes/1 -> Mux1/2
  Selector2/1 -> Mux/1
  Vr Roll Axes/1 -> Mux/2
  Euler Angles/1 -> Selector2/1, Selector1/1, Selector/1
  Quaternion Multiplication (Pitch & Yaw)/1 -> Quaternion Multiplication (Roll)/1

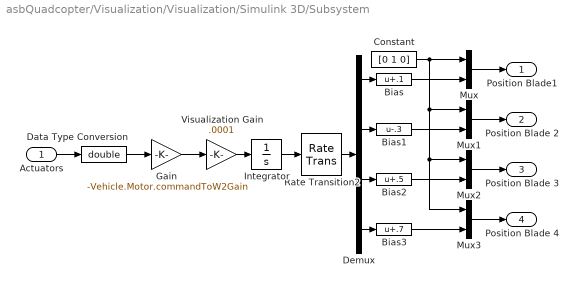
== system asbQuadcopter/Visualization/Visualization/Simulink 3D/Subsystem ==
  Actuators : Inport
  Bias : Bias  Bias=.1
  Bias1 : Bias  Bias=-.3
  Bias2 : Bias  Bias=.5
  Bias3 : Bias  Bias=.7
  Constant : Constant  Value=[0 1 0]
  Data Type Conversion : DataTypeConversion  OutDataTypeStr=double
  Demux : Demux
  Gain : Gain  Gain=-Vehicle.Motor.commandToW2Gain
  Integrator : Integrator  InitialCondition="[.1  .2 -.3 -.4]"  WrapState=on  WrappedStateUpperValue=2*pi  WrappedStateLowerValue=-2*pi
  Mux{,1..3} (4 alike) : Mux  Inputs=2
  Rate Transition2 : RateTransition
  Visualization Gain : Gain  Gain=.0001
  Position Blade1 : Outport
  Position Blade 2 : Outport  Port=2
  Position Blade 3 : Outport  Port=3
  Position Blade 4 : Outport  Port=4
  wires:
  Bias3/1 -> Mux3/2
  Mux3/1 -> Position Blade 4/1
  Bias1/1 -> Mux1/2
  Bias2/1 -> Mux2/2
  Demux/2 -> Bias1/1
  Visualization Gain/1 -> Integrator/1
  Constant/1 -> Mux3/1, Mux2/1, Mux1/1, Mux/1
  Mux1/1 -> Position Blade 2/1
  Mux2/1 -> Position Blade 3/1
  Data Type Conversion/1 -> Gain/1
  Integrator/1 -> Rate Transition2/1
  Mux/1 -> Position Blade1/1
  Gain/1 -> Visualization Gain/1
  Demux/3 -> Bias2/1
  Bias/1 -> Mux/2
  Actuators/1 -> Data Type Conversion/1
  Demux/4 -> Bias3/1
  Rate Transition2/1 -> Demux/1
  Demux/1 -> Bias/1

== system asbQuadcopter/Visualization/Visualization/Simulink 3D/Euler to VR/Axis Angle Vector ==
  e0 : Inport
  2 : Gain  Gain=2  SaturateOnIntegerOverflow=on  OutDataTypeStr=Inherit: Same as input  ParamDataTypeStr=Inherit: Same as input
  Constant : Constant  Value=1e-6
  Demux : Demux  Outputs=[1 3 ]
  Mux : Mux  Inputs=2
  Product : Product  Inputs=*/  SaturateOnIntegerOverflow=on  InputSameDT=on  OutDataTypeStr=Inherit: Same as first input
  Switch : Switch  Criteria=u2 ~= 0
  Trigonometric Function : Trigonometry
  Trigonometric Function2 : Trigonometry  Operator=acos
  e0_norm : Outport
  wires:
  Demux/1 -> Trigonometric Function2/1
  Demux/2 -> Product/1
  Mux/1 -> e0_norm/1
  Product/1 -> Mux/1
  2/1 -> Mux/2
  Trigonometric Function/1 -> Switch/1, Switch/2
  Trigonometric Function2/1 -> Trigonometric Function/1, 2/1
  e0/1 -> Demux/1
  Constant/1 -> Switch/3
  Switch/1 -> Product/2

== system asbQuadcopter/Visualization/Visualization/Simulink 3D/Euler to VR/Quaternion Normalization ==
  e0 : Inport
  1/2 : Gain  Gain=1/2  SaturateOnIntegerOverflow=on  OutDataTypeStr=Inherit: Same as input  ParamDataTypeStr=Inherit: Same as input
  Demux : Demux  Outputs=[1 3]
  Mux : Mux  Inputs=2
  Product : Product  SaturateOnIntegerOverflow=on  InputSameDT=on  OutDataTypeStr=Inherit: Same as first input
  Trigonometric Function : Trigonometry
  Trigonometric Function1 : Trigonometry  Operator=cos
  e0_norm : Outport
  wires:
  Trigonometric Function1/1 -> Mux/1
  Demux/2 -> Product/2
  Demux/1 -> 1/2/1
  Mux/1 -> e0_norm/1
  Product/1 -> Mux/2
  Trigonometric Function/1 -> Product/1
  1/2/1 -> Trigonometric Function1/1, Trigonometric Function/1
  e0/1 -> Demux/1

== system asbQuadcopter/Visualization/Visualization/Simulink 3D/Euler to VR/Quaternion Normalization1 ==
  e0 : Inport
  1/2 : Gain  Gain=1/2  SaturateOnIntegerOverflow=on  OutDataTypeStr=Inherit: Same as input  ParamDataTypeStr=Inherit: Same as input
  Demux : Demux  Outputs=[1 3]
  Mux : Mux  Inputs=2
  Product : Product  SaturateOnIntegerOverflow=on  InputSameDT=on  OutDataTypeStr=Inherit: Same as first input
  Trigonometric Function : Trigonometry
  Trigonometric Function1 : Trigonometry  Operator=cos
  e0_norm : Outport
  wires:
  e0/1 -> Demux/1
  1/2/1 -> Trigonometric Function/1, Trigonometric Function1/1
  Trigonometric Function/1 -> Product/1
  Product/1 -> Mux/2
  Mux/1 -> e0_norm/1
  Demux/1 -> 1/2/1
  Demux/2 -> Product/2
  Trigonometric Function1/1 -> Mux/1

== system asbQuadcopter/Visualization/Visualization/Simulink 3D/Euler to VR/Quaternion Normalization2 ==
  e0 : Inport
  1/2 : Gain  Gain=1/2  SaturateOnIntegerOverflow=on  OutDataTypeStr=Inherit: Same as input  ParamDataTypeStr=Inherit: Same as input
  Demux : Demux  Outputs=[1 3]
  Mux : Mux  Inputs=2
  Product : Product  SaturateOnIntegerOverflow=on  InputSameDT=on  OutDataTypeStr=Inherit: Same as first input
  Trigonometric Function : Trigonometry
  Trigonometric Function1 : Trigonometry  Operator=cos
  e0_norm : Outport
  wires:
  Trigonometric Function1/1 -> Mux/1
  Demux/2 -> Product/2
  Demux/1 -> 1/2/1
  Mux/1 -> e0_norm/1
  Product/1 -> Mux/2
  Trigonometric Function/1 -> Product/1
  1/2/1 -> Trigonometric Function1/1, Trigonometric Function/1
  e0/1 -> Demux/1
